simulink model "slip_simulink"  (R2015b)
settings: Solver=VariableStepAuto  StartTime=0.0  StopTime=10.0  RelTol=1e-3
libraries: simulink x1
settings Model: Creator=robots  LastModifiedBy=robots

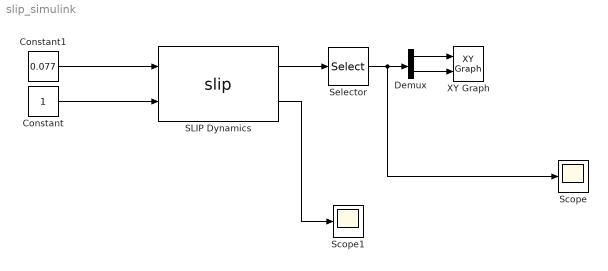
== system slip_simulink ==
  Constant : Constant
  Constant1 : Constant  Value=0.077
  Demux : Demux  Outputs=2
  SLIP Dynamics : M-S-Function  FunctionName=slip  Parameters=m, k, b, g, Y0  mask{m=10, k=1000, b=10, g=9.81, Y0=[0 1.2 0.1 0]}
      mask prompts: m "Mass"; k "Stiffness"; b "Damping"; g "Gravity"; Y0 "Initial conditions"
      mask Display:
      | port_label('input', 1, 'angle')
      | port_label('input', 2, 'length')
      | port_label('output', 1, 'states')
      | port_label('output', 2, 'phase')
  Scope : Scope
  Scope1 : Scope
  Selector : Selector  InputPortWidth=9  IndexOptions=Index vector (dialog)  Indices=[1 2]  OutputSizes=1
  XY Graph : simulink/Sinks/XY Graph  xmin=-5  xmax=10  ymin=-1  ymax=3  st=-1
  wires:
  Constant/1 -> SLIP Dynamics/2
  Constant1/1 -> SLIP Dynamics/1
  SLIP Dynamics/1 -> Selector/1
  Selector/1 -> Scope/1, Demux/1
  Demux/1 -> XY Graph/1
  Demux/2 -> XY Graph/2
  SLIP Dynamics/2 -> Scope1/1
